simulink model "fishball_scanner"  (R2026a)
settings: Solver=FixedStepDiscrete  StopTime=19.9111111
undefined symbols (not defined in the file or in its folder): repelem
libraries: simulink x1
settings Model: Creator=matthieu  LastModifiedBy=matthieu

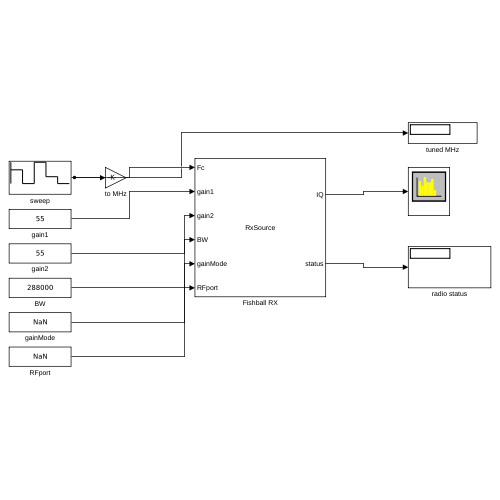
[thumbnail: Simulink's stored preview of the top-level diagram]
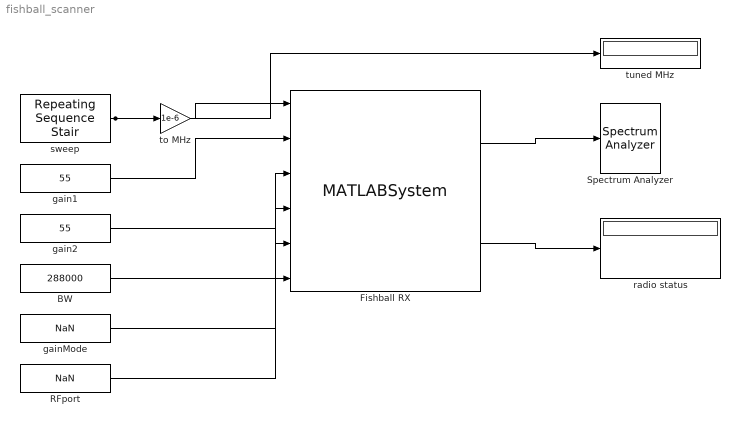
== system fishball_scanner ==
  BW : Constant  Value=288000
  Fishball RX : MATLABSystem  System=fishball.RxSource  ChannelMapping=RX1  CenterFrequency=88000000  RFBandwidth=0  RFPort=A Balanced  GainSource=Manual  Gain=55  BasebandSampleRate=288000  FabricDecimation=8  SamplesPerFrame=4096  EnableQuadratureTracking=on  EnableRFDCTracking=on  EnableBasebandDCTracking=on  EnableRxFIR=off  ControlPorts=all  StatusUpdatePeriod=1  SimulateUsing=Interpreted execution
      mask Type: fishball.RxSource
  RFport : Constant  Value=NaN
  Spectrum Analyzer : SpectrumAnalyzer  WindowInvariantSamplesPerUpdate=on
  gain1 : Constant  Value=55
  gain2 : Constant  Value=55
  gainMode : Constant  Value=NaN
  radio status : Display
  sweep : simulink/Sources/Repeating Sequence Stair  OutValues=repelem(88000000:288000:108000000, 20)  tsamp=4096/288000  OutMin=[]  OutMax=[]  OutDataTypeStr=double  OutputDataTypeScalingMode=double  OutDataType=fixdt(0,8)  ConRadixGroup=Best Precision: Vector-wise  OutScaling=2^-12
  to MHz : Gain  Gain=1e-6
  tuned MHz : Display
  wires:
  sweep/1 -> Fishball RX/1, to MHz/1
  gain1/1 -> Fishball RX/2
  gain2/1 -> Fishball RX/3
  BW/1 -> Fishball RX/4
  gainMode/1 -> Fishball RX/5
  RFport/1 -> Fishball RX/6
  Fishball RX/1 -> Spectrum Analyzer/1
  Fishball RX/2 -> radio status/1
  to MHz/1 -> tuned MHz/1
